simulink library "CommercialVehicleLibrary2G"  (R2021a)
settings: Solver=VariableStepAuto  StartTime=0.0  StopTime=10.0  RelTol=1e-3
values from neighbouring files (symbols this model uses):
  brake_input = [0   tmax ... (first row only)    [init_vehicle.m]    (also in run_Circle.m = [0  tmax; run_Coastdown.m = [0  2  tmax; run_DoubleLaneChangeDriver.m = [0   2  tmax; run_MaxAcc.m = [0  2  tmax)
  pose_t0 = [0 0 0 0]    [init_vehicle.m]    (also in run_Circle.m; run_Coastdown.m; run_DoubleLaneChangeDriver.m; run_MaxAcc.m)
  rdfname = 'TNO_FlatRoad.rdf'    [run_Circle.m]    (also in run_Coastdown.m; run_DoubleLaneChangeDriver.m; run_MaxAcc.m; run_Rollover.m)
  rdfname_inner = 'TNO_FlatRoad.rdf'    [run_Circle.m]    (also in run_Coastdown.m; run_DoubleLaneChangeDriver.m; run_MaxAcc.m; run_Rollover.m)
  steer_input = [0  tmax ... (first row only)    [init_vehicle.m]    (also in run_Circle.m = [0  2   10     13       tmax; run_Coastdown.m = [0 tmax; run_DoubleLaneChangeDriver.m = [0 tmax; run_MaxAcc.m = [0 tmax)
  throttle_input = [0         tmax ... (first row only)    [init_vehicle.m]    (also in run_Circle.m; run_Coastdown.m = [0        10         10.0001 tmax; run_DoubleLaneChangeDriver.m = [0        tmax; run_MaxAcc.m = [0        tmax)
  Vx = 0    [init_vehicle.m]    (also in run_Circle.m = Vx_kmh/3.6; run_Coastdown.m = Vx_kmh/3.6; run_DoubleLaneChangeDriver.m = Vx_kmh/3.6; run_MaxAcc.m)
  Vx_input = [0  tmax ... (first row only)    [init_vehicle.m]    (also in run_Circle.m; run_Coastdown.m = [0 tmax; run_DoubleLaneChangeDriver.m = [0 tmax; run_MaxAcc.m = [0 tmax)
undefined symbols (not defined in the file or in its folder): Drive, Floor, Fzstat, Fzstat1, Fzstat3, l, l_load1, l_load2, lbar, mass_load1, mass_load2, psi_semitrailer, rho, rim_Ixx, rim_Iyy, rim_mass, Steer, steer_path, tpfname, X, x_torsion, xcg, xcg1, xcg2, xcg_front, xcg_rear, xdrive1, xload1, xload2, xpos1, xref, xrev1, Xt0, Y, Yt0, Z
libraries: sm_lib x291, $bdroot x157, nesl_utility x143, vrlib x1
(part 1 of 12)
settings Model: Creator=ajayk  LastModifiedBy=ajayk
settings SolverCC: AlgebraicLoopSolver=TrustRegion
settings DebuggingCC: SFMachineParentedDataDiag=warning

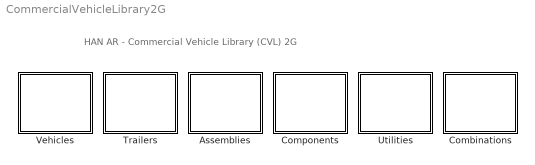
== system CommercialVehicleLibrary2G ==
  note: HAN AR - Commercial Vehicle Library (CVL) 2G
  Assemblies : Subsystem
      mask Display: disp('Assemblies')
  Combinations : Subsystem
      mask Display: disp('Combinations')
  Components : Subsystem
      mask Display: disp('Components')
  Trailers : Subsystem
      mask Display: disp('Trailers')
  Utilities : Subsystem
      mask Display: disp('Utilities')
  Vehicles : Subsystem
      mask Display: disp('Vehicles')

== system CommercialVehicleLibrary2G/Assemblies ==
  note: Axles
  note: Loads
  Cabin : Subsystem  mask(cabin with coil/air suspension){xref=xref+1.10, zref=1.20}
      mask prompts: xref "global X-coordinate cabin tip point [m]"; zref "global Z-coordinate cabin tip point [m]"
      mask Display: disp('Cabin')
  Dolly axle : Subsystem  mask(Axle with single tyres){xpos=0.7, tpfname='truck3.tpf', rdfname=rdfname, Vx=Vx, Fzstat=Fzstat}
      mask prompts: xpos "global X-coordinate wheelcentre [m]"; tpfname "tyre property file name [string]"; rdfname "road data file name  [string]"; Vx "initial velocity Vx [m/s]"; Fzstat "initial vertical axle load [N]"
      mask init:
      | Rtyre     = 0.546;
      | Cztyre    = 1.35e+006;
      | tyre_mass = 70;
      | 
      | zpos   =Rtyre - 0.5*Fzstat/Cztyre;
      | 
      | % dimensions
      | tw =2.0;  % [m], track_width
      | yd =1.0;  % [m], Y-distance bewteen dampers
      | ys =1.0;  % [m], Y-distance bewteen springs 
      | zrc=0.2;  % [m], height of roll centre wrt axle 
      |    
      | % damping/stiffness
      | Kspring = 394000;  % [N/m], spring stiffness (two per axle!)
      | Bdamper =  20000;  % [Ns/m] damper constant (two per axle!)
      | Kroll   =1516000;  % [Nm/rad] roll stiffness 
      |    
      | % mass/inertia
      | axle_mass = 400;  % [kg]
      | axle_Ixx  = 200; % [kgm2]
      | axle_Iyy  =  10;   % [kgm2]
      | axle_Izz  = 200; % [kgm2]
      |    
      | rim_mass= 55; % [kg]
      | rim_Ixx =  4; % [kgm2]
      | rim_Iyy =  6; % [kgm2] (including rotational inertia brake disk)
      | 
      | ld = 0.3;                     % loaded spring/damper length
      | ls = ld + 0.5*(Fzstat - 9.81*(axle_mass + 2*tyre_mass + 2*rim_mass))/Kspring;  % spring unloaded length
  Drive axle : Subsystem  mask(Driven axle with double tyres){xpos=xdrive1, tpfname='truck1.tpf', rdfname=rdfname, rdfname_inner=rdfname_inner, Vx=Vx, Fzstat=Fzstat3}
      mask prompts: xpos "global X-coordinate wheelcentre [m]"; tpfname "tyre property file name [string]"; rdfname "road data file name  [string]"; rdfname_inner "road data file name (inner)  [string]"; Vx "initial velocity Vx [m/s]"; Fzstat "initial vertical axle load [N]"
      mask init:
      | Rtyre     = 0.548;
      | Cztyre    = 1.13e+006;
      | tyre_mass = 62.7;
      | 
      | zpos = Rtyre - 0.25*Fzstat/Cztyre;
      | 
      | tw  =2.15;    % [m], track_width outer tyres
      | ywhl=0.35;   % [m], distance between double tyres
      | yd  =1.00;    % [m], Y-distance bewteen dampers
      | ys  =0.75;    % [m], Y-distance bewteen springs
      | zrc =0.30;   % [m], height of roll centre wrt axle centre 
      | 
      | % damping/stiffness
      | Kspring = 320000;    % [N/m], spring stiffness  (two per axle!)
      | Bdamper =  15000;    % [Ns/m], damper constant  (two per axle!)
      | Kroll   = 500000;    % [Nm/rad] roll stiffness 
      | 
      | % mass/inertia
      | axle_mass =1000;     % [kg] (excl. wheels/tyres!)
      | axle_Ixx  = 380;     % [kgm2]
      | axle_Iyy  =  10;     % [kgm2]
      | axle_Izz  = 380;     % [kgm2]
      |    
      | %rim
      | rim_mass= 50;        % [kg]
      | rim_Ixx =  3;        % [kgm2]
      | rim_Iyy =  5;        % [kgm2] (including rotational inertia brake disk)
      | 
      | ld = 0.3;            % loaded spring/damper length
      | ls = ld + 0.5*(Fzstat - 9.81*(axle_mass + 4*tyre_mass + 4*rim_mass))/Kspring;  % spring unloaded length
  Driveline : Subsystem  mask(Engine+gearbox){xref=xref-0.162, zref=0.58, param=DAF XEC + TC-Tronic (355 kW/2100 Nm)}
      mask prompts: xref "global X-coordinate engine ref. point [m]"; zref "global Z-coordinate engine ref. point [m]"; param "parameters"
      mask init:
      | % engine/gearbox: DAF XE355C / ZF 16S221
      | eng_power         = 355000;  % 355 kW
      | max_engine_torque = 2100;    % [Nm]
      | max_revs_rpm      = 1900;    % [rpm]
      | first_gear_ratio  = 16.41;   % [-]
      | final_drive_ratio =  3.07;   % [-]
      |  
      | % engine + gearbox mass (XEC +TC-tronic, DAF 51051/03-042 R. Liebrechts)
      | driveline_mass= 1800;       %[kg]
      | Ixx =  100;       %[kgm2]
      | Iyy =  900;       %[kgm2]
      | Izz =  900;       %[kgm2]
      | yrot=   0;        %[rad] rotation about Y-axis of inertial frame
      | xcg =  -0.25;     %[m], X-coordinate CG wrt rear engine mount ref. point
      | zcg =   0.30;     %[m], Z-coordinate CG wrt rear engine mount ref. point
      |  
      | omega_max=2*pi*max_revs_rpm/60;
      mask TypeOptions param: DAF XEC + TC-Tronic (355 kW/2100 Nm)
  Driver : Subsystem
  Steer axle : Subsystem  mask(Axle with single tyres and steering system){xpos=xref, tpfname='truck2b2.tpf', rdfname=rdfname, Vx=Vx, Fzstat=Fzstat1}
      mask prompts: xpos "global X-coordinate wheelcentre [m]"; tpfname "tyre property file name [string]"; rdfname "road data file name  [string]"; Vx "initial velocity Vx [m/s]"; Fzstat "initial vertical axle load [N]"
      mask init:
      | Rtyre    = 0.548;
      | Cztyre   = 1.19e+006;
      | tyre_mass= 62.7;
      | 
      | zpos=Rtyre - 0.5*Fzstat/Cztyre;
      | 
      | steerratio = 20; %[-], ratio steering wheel - front wheels
      |  
      | % dimensions
      | tw =2.0; 	% [m], track_width
      | zrc=0;    	% [m], height of roll centre wrt axle centerline   
      | yd =1.0; 	% [m], Y-distance bewteen dampers 
      | ys =0.85; 	% [m], Y-distance bewteen springs
      | 
      | % stiffness/damping
      | Kspring = 300000;  	% [N/m], spring stiffness (two per axle!)
      | Bdamper =  15000;  	% [Ns/m] damper constant  (two per axle!)
      | Kroll   = 200000;  	% [Nm/rad], roll stiffness 
      |    
      | % mass/inertia   
      | axle_mass = 475;    % [kg] (excl. wheels/tyres!)
      | axle_Ixx  = 200;	% [kgm2]
      | axle_Iyy  = 5;      % [kgm2]
      | axle_Izz  = 200;	% [kgm2]
      |    
      | %rim mass
      | rim_mass= 50; 	% [kg]
      | rim_Ixx =  3; 	% [kgm2]
      | rim_Iyy =  5; 	% [kgm2] (including rotational inertia brake disk)
      | 
      | ld = 0.3;       % loaded spring/damper length
      | ls = ld + 0.5*(Fzstat - 9.81*(axle_mass + 2*tyre_mass + 2*rim_mass))/Kspring;  % spring unloaded length
  Trailer axle : Subsystem  mask(Axle with single tyres){xpos=xpos1-xcg, tpfname='truck3.tpf', rdfname=rdfname, Vx=Vx, Fzstat=Fzstat}
      mask prompts: xpos "global X-coordinate wheelcentre [m]"; tpfname "tyre property file name [string]"; rdfname "road data file name  [string]"; Vx "initial velocity Vx [m/s]"; Fzstat "initial vertical axle load [N]"
      mask init: same as CommercialVehicleLibrary2G/Assemblies/Dolly axle
  Trailer load center : Subsystem  mask{xload=xload1, zload=1.3, mass_load=mass_load1, l_load=l_load1, w=2.5, rho=rho}
      mask prompts: xload "Global X-coordinate Center of Load [m]"; zload "Global Z-coordinate Application of Load [m]"; mass_load "mass [kg]"; l_load "length [m]"; w "width [m]"; rho "density [kg/m3]"
      mask init:
      | h=(mass_load)/(rho*w*(l_load));
      | zcg=0.5*h;
      | Ixx=(mass_load)*(w*w+h*h)/12;
      | Iyy=(mass_load)*((l_load)*(l_load)+h*h)/12;
      | Izz=(mass_load)*((l_load)*(l_load)+w*w)/12;
      mask Display: disp('Trailer center load ')
  Trailer load front : Subsystem  mask{xload=xload1, zload=1.3, mass_load=mass_load1, l_load=l_load1, w=2.5, rho=rho}
      mask prompts: xload "Global X-coordinate Center of Load [m]"; zload "Global Z-coordinate Application of Load [m]"; mass_load "mass [kg]"; l_load "length [m]"; w "width [m]"; rho "density [kg/m3]"
      mask init:
      | h=(mass_load)/(rho*w*(l_load));
      | zcg=0.5*h;
      | Ixx=(mass_load)*(w*w+h*h)/12;
      | Iyy=(mass_load)*((l_load)*(l_load)+h*h)/12;
      | Izz=(mass_load)*((l_load)*(l_load)+w*w)/12;
      mask Display: disp('Trailer front load ')
  Trailer load rear : Subsystem  mask{xload=xload2, zload=1.3, mass_load=mass_load2, l_load=l_load2, w=2.5, rho=rho}
      mask prompts: xload "Global X-coordinate Center of Load [m]"; zload "Global Z-coordinate Application of Load [m]"; mass_load "mass [kg]"; l_load "length [m]"; w "width [m]"; rho "density [kg/m3]"
      mask init:
      | h=(mass_load)/(rho*w*(l_load));
      | zcg=0.5*h;
      | Ixx=(mass_load)*(w*w+h*h)/12;
      | Iyy=(mass_load)*((l_load)*(l_load)+h*h)/12;
      | Izz=(mass_load)*((l_load)*(l_load)+w*w)/12;
      mask Display: disp('Trailer rear load ')
  Truck load : Subsystem  mask{xload=xload2, zload=1.3, mass_load=mass_load2, l_load=l_load2, w=2.5, rho=rho}
      mask prompts: xload "Global X-coordinate Center of Load [m]"; zload "Global Z-coordinate Application of Load [m]"; mass_load "mass [kg]"; l_load "length [m]"; w "width [m]"; rho "density [kg/m3]"
      mask init:
      | h=(mass_load)/(rho*w*(l_load));
      | zcg=0.5*h;
      | Ixx=(mass_load)*(w*w+h*h)/12;
      | Iyy=(mass_load)*((l_load)*(l_load)+h*h)/12;
      | Izz=(mass_load)*((l_load)*(l_load)+w*w)/12;
      mask Display: disp('Truck load ')

== system CommercialVehicleLibrary2G/Combinations ==
  note: Custom Combinations
  note: LZV Combinations
  LZV_A : Subsystem
      mask Display: disp('LZV - A')
  LZV_B : Subsystem
      mask Display: disp('LZV - B ')
  LZV_C : Subsystem
      mask Display: disp('LZV - C')
  LZV_D : Subsystem
      mask Display: disp('LZV - D')
  LZV_E : Subsystem
      mask Display: disp('LZV - E')
  LZV_F : Subsystem
      mask Display: disp('LZV - F')
  LZV_G : Subsystem
      mask Display: disp('LZV - G')
  "Tractor_semitrailer " : Subsystem
      mask Display: disp('Tractor + Semitrailer')
  Truck_dbtrailer : Subsystem
      mask Display: disp('Truck + DbTrailer')
  Truck_trailer : Subsystem
      mask Display: disp('Truck + Trailer')

== system CommercialVehicleLibrary2G/Components ==
  5th Wheel Joint : Subsystem
      mask Display: disp('5th Wheel Joint')
  Brake/Wheel_bearing : Subsystem  mask{Vx=Vx, radius=0.53}
      mask prompts: Vx "forward velocity (m/s)"; radius "tyre radius (m)"
  Braking system : Subsystem
  "Drawbar joint " : Subsystem
      mask Display: disp('Drawbar joint')
  MF Tyre L : Subsystem  Tag=SimMechanics Wheel + tyre  mask(SimMechanics_tyre){idtyre=1, inertia=[rim_mass rim_Ixx rim_Iyy], tpfname=tpfname, rdfname=rdfname, side_mode=(1xxx) left, cnt_mode=(x1xx) smooth road, dyn_mode=(xx1x) relaxation behaviour, mf_mode=(xxx4) combined, use_mode=1e8, disp_debug=off}
      mask prompts: idtyre "Tyre ID [integer]"; inertia "Rim inertia [3x real] mass (kg) Ixx Iyy (kgm2)"; tpfname "Tyre properties [string or struct]"; rdfname "Road data file [string]"; side_mode "Tyre side            :"; cnt_mode "Contact method :"; dyn_mode "Dynamics           :"; mf_mode "Slip forces          :"; use_mode "Optional: use mode (overrides pop-up) [current selection: 1114]"; disp_debug "Display debug messages"
      mask help:
      | Wheel + tyre model to be used in combination with the SimMechanics multibody toolbox.
      |
      | Tyre model version: MF-Tyre/MF-Swift 6.2
      | © 1996-2013 TNO, Helmond, The Netherlands
      |
      | MODIFIED VERSION by TU/e! (Igo Besselink)
      mask init:
      | % initialize parameters
      | % (required to overcome a bug in MATLAB 2006a: errors in a mask are not displayed,
      | %  and simulation is not ended. This check is carried out in s-function 
      | %  'chech_inertia_parameters' in the subsystem)
      | radius     = 1;
      | width      = 1;
      | belt_mass  = 1;
      | belt_Ixx   = 1;
      | belt_Iyy   = 1;
      | tyre_mass  = 1;
      | tyre_Ixx   = 1;
      | tyre_Iyy   = 1;
      | mass = 1;
      | Imat = [1 0 0; 0 1 0; 0 0 1];
      | 
      | % switch between tpf file or struct
      | if ischar(tpfname)
      |     typarr=zeros(300,1);
      |     tpfname_dummy=tpfname;
      |     if ~exist(tpfname_dummy)
      |         error('Tyre property file does not exist')
      |     end
      | elseif isstruct(tpfname)
      |     typarr=tno_tpf_struct2array(tpfname,idtyre);
      |     tpfname_dummy='';
      | else
      |     typarr=zeros(300,1);
      |     tpfname_dummy='';
      |     error(['Mask parameter ''Tyre property file'' should be supplied as string or structure for tyre ' num2str(idtyre)])
      | end
      | if ~exist(rdfname) && ~strcmp(rdfname,'')
      |     error('Road data file does not exist')
      | end
      | 
      | %initialisation script for SimMechanics
      | idroad=1;
      | 
      | %rim inertia as specified by the user in the GUI
      | rim_mass = inertia(1);
      | rim_Ixx  = inertia(2);
      | rim_Iyy  = inertia(3);
      | 
      | % check the use_mode of the model
      | if (abs(use_mode) > 4535 )
      |   iswtch=1000*side_mode+100*cnt_mode+10*(dyn_mode-1)+(mf_mode-1);
      | else
      |   iswtch=use_mode;
      | end
      | 
      | %get tyre inertia parameters from the tyre property file
      | if ischar(tpfname)
      |     [x,typarr]=dteval(tpfname_dummy,[1 2 3 4 5 6],1);
      | end
      | radius     = typarr(7);
      | width      = typarr(8);
      | belt_mass  = typarr(164);
      | belt_Ixx   = typarr(195);
      | belt_Iyy   = typarr(162);
      | tyre_mass  = typarr(190);
      | tyre_Ixx   = typarr(191);
      | tyre_Iyy   = typarr(192);
      | 
      | % display the use_mode of the model
      | if (disp_debug) disp(['Delft-Tyre ' num2str(idtyre) ' -> use_mode=' num2str(iswtch) ]); end
      | 
      | % check and calculate inertia of the rim_body
      | if  ( rim_mass <= 0 | rim_Ixx <= 0 | rim_Iyy <= 0 | tyre_mass <= 0 | tyre_Ixx <= 0 | tyre_Iyy <= 0 | belt_mass <= 0 | belt_Ixx <= 0 | belt_Iyy <= 0 )
      |   error('initialisation calculation results in a negative mass and/or inertia!') 
      |   disp_debug=1;
      | end
      | if  ( tyre_mass <= belt_mass | tyre_Ixx <= belt_Ixx | tyre_Iyy <= belt_Iyy  )
      |   error('initialisation calculation error: tyre belt mass/inertia > tyre mass/inertia!') 
      |   disp_debug=1;
      | end
      | 
      | if (disp_debug) 
      |   msg=[' wheel mass = ',num2str(rim_mass+tyre_mass),' kg'];
      |   disp(msg);
      |   msg=[' wheel Ixx  = ',num2str(rim_Ixx+tyre_Ixx),' kgm2'];
      |   disp(msg);
      |   msg=[' wheel Iyy  = ',num2str(rim_Iyy+tyre_Iyy),' kgm2'];
      |   disp(msg);
      |   msg=[' tyre mass  = ',num2str(tyre_mass),' kg (belt mass = ',num2str(belt_mass),' kg)' ];
      |   disp(msg);
      |   msg=[' tyre Ixx   = ',num2str(tyre_Ixx) ,' kgm2 (belt Ixx  = ',num2str(belt_Ixx) ,' kgm2)'];
      |   disp(msg);
      |   msg=[' tyre Iyy   = ',num2str(tyre_Iyy) ,' kgm2 (belt Iyy  = ',num2str(belt_Iyy) ,' kgm2)'];
      |   disp(msg);
      | end
      | 
      | % calculate the mass of the wheelbody in the MBS environment 
      | %   normally           : rim + tyre
      | %   rigid ring dynamics: rim + part of tyre (and separate rigid body inside tyre model)
      | dynmod=iswtch-100*floor(iswtch/100);
      | if (dynmod/10 >= 3) 
      |   %rigid ring dynamics switched on
      |   wheelbody_mass = rim_mass + tyre_mass - belt_mass;
      |   wheelbody_Ixx  = rim_Ixx  + tyre_Ixx  - belt_Ixx;
      |   wheelbody_Iyy  = rim_Iyy  + tyre_Iyy  - belt_Iyy;
      | else
      |   %rigid ring dynamics switched off
      |   wheelbody_mass = rim_mass + tyre_mass;
      |   wheelbody_Ixx  = rim_Ixx  + tyre_Ixx;
      |   wheelbody_Iyy  = rim_Iyy  + tyre_Iyy;
      | end
      | 
      | mass = wheelbody_mass;
      | Imat = [wheelbody_Ixx 0 0; 0 wheelbody_Iyy 0; 0 0 wheelbody_Ixx];
      | 
      | fliplr = 0;
      | % CHANGE GEOMETRY ORIENTATION IF WHEEL IS ON RIGHT SIDE
      | if (side_mode == 2)
      |     fliplr=1;
      |     %disp(['Tyre ID = ' num2str(idtyre) ', fliplr = ' num2str(fliplr)]);
      | end
      mask Help: eval('DTOpenHelp(506)')
      mask TypeOptions side_mode: (1xxx) left | (2xxx) right | (3xxx) symmetric
      mask Callback side_mode:
      | promtstr = get_param(gcb,'MaskPromptString');
      | index = find(double(promtstr)==124);
      | maskval = get_param(gcb,'MaskValues');
      | new_mode = [maskval{5}(2) maskval{6}(3) maskval{7}(4) maskval{8}(5)];
      | newpromtstr = [promtstr(1:index(8)) ['Optional: use mode (overrides pop-up) [current selection: ' new_mode ']'] promtstr(index(9):end)];
      | set_param(gcb,'MaskPromptString',newpromtstr);
      mask TypeOptions cnt_mode: (x1xx) smooth road | (x2xx) smooth road (motorcycle: circular cross section) | (x3xx) moving road | (x4xx) 2D short wavelength road contact | (x5xx) 3D short wavelength road contact
      mask Callback cnt_mode:
      | promtstr = get_param(gcb,'MaskPromptString');
      | index = find(double(promtstr)==124);
      | maskval = get_param(gcb,'MaskValues');
      | new_mode = [maskval{5}(2) maskval{6}(3) maskval{7}(4) maskval{8}(5)];
      | newpromtstr = [promtstr(1:index(8)) ['Optional: use mode (overrides pop-up) [current selection: ' new_mode ']'] promtstr(index(9):end)];
      | set_param(gcb,'MaskPromptString',newpromtstr);
      mask TypeOptions dyn_mode: (xx0x) steady-state | (xx1x) relaxation behaviour | (xx2x) relaxation behaviour - non-linear | (xx3x) rigid ring | (xx4x) rigid ring + initial statics
      mask Callback dyn_mode:
      | promtstr = get_param(gcb,'MaskPromptString');
      | index = find(double(promtstr)==124);
      | maskval = get_param(gcb,'MaskValues');
      | new_mode = [maskval{5}(2) maskval{6}(3) maskval{7}(4) maskval{8}(5)];
      | newpromtstr = [promtstr(1:index(8)) ['Optional: use mode (overrides pop-up) [current selection: ' new_mode ']'] promtstr(index(9):end)];
      | set_param(gcb,'MaskPromptString',newpromtstr);
      mask TypeOptions mf_mode: (xxx0) none | (xxx1) longitudinal | (xxx2) lateral | (xxx3) uncombined | (xxx4) combined | (xxx5) combined+turnslip
      mask Callback mf_mode:
      | promtstr = get_param(gcb,'MaskPromptString');
      | index = find(double(promtstr)==124);
      | maskval = get_param(gcb,'MaskValues');
      | new_mode = [maskval{5}(2) maskval{6}(3) maskval{7}(4) maskval{8}(5)];
      | newpromtstr = [promtstr(1:index(8)) ['Optional: use mode (overrides pop-up) [current selection: ' new_mode ']'] promtstr(index(9):end)];
      | set_param(gcb,'MaskPromptString',newpromtstr);
  MF Tyre R : Subsystem  Tag=SimMechanics Wheel + tyre  mask(SimMechanics_tyre){idtyre=2, inertia=[rim_mass rim_Ixx rim_Iyy], tpfname=tpfname, rdfname=rdfname, side_mode=(2xxx) right, cnt_mode=(x1xx) smooth road, dyn_mode=(xx1x) relaxation behaviour, mf_mode=(xxx4) combined, use_mode=1e8, disp_debug=off}
      mask prompts: idtyre "Tyre ID [integer]"; inertia "Rim inertia [3x real] mass (kg) Ixx Iyy (kgm2)"; tpfname "Tyre properties [string or struct]"; rdfname "Road data file [string]"; side_mode "Tyre side            :"; cnt_mode "Contact method :"; dyn_mode "Dynamics           :"; mf_mode "Slip forces          :"; use_mode "Optional: use mode (overrides pop-up) [current selection: 2114]"; disp_debug "Display debug messages"
      mask help:
      | Wheel + tyre model to be used in combination with the SimMechanics multibody toolbox.
      |
      | Tyre model version: MF-Tyre/MF-Swift 6.2
      | © 1996-2013 TNO, Helmond, The Netherlands
      |
      | MODIFIED VERSION by TU/e! (Igo Besselink)
      mask init: same as CommercialVehicleLibrary2G/Components/MF Tyre L
      mask Help: eval('DTOpenHelp(506)')
      mask TypeOptions side_mode: (1xxx) left | (2xxx) right | (3xxx) symmetric
      mask Callback side_mode:
      | promtstr = get_param(gcb,'MaskPromptString');
      | index = find(double(promtstr)==124);
      | maskval = get_param(gcb,'MaskValues');
      | new_mode = [maskval{5}(2) maskval{6}(3) maskval{7}(4) maskval{8}(5)];
      | newpromtstr = [promtstr(1:index(8)) ['Optional: use mode (overrides pop-up) [current selection: ' new_mode ']'] promtstr(index(9):end)];
      | set_param(gcb,'MaskPromptString',newpromtstr);
      mask TypeOptions cnt_mode: (x1xx) smooth road | (x2xx) smooth road (motorcycle: circular cross section) | (x3xx) moving road | (x4xx) 2D short wavelength road contact | (x5xx) 3D short wavelength road contact
      mask Callback cnt_mode:
      | promtstr = get_param(gcb,'MaskPromptString');
      | index = find(double(promtstr)==124);
      | maskval = get_param(gcb,'MaskValues');
      | new_mode = [maskval{5}(2) maskval{6}(3) maskval{7}(4) maskval{8}(5)];
      | newpromtstr = [promtstr(1:index(8)) ['Optional: use mode (overrides pop-up) [current selection: ' new_mode ']'] promtstr(index(9):end)];
      | set_param(gcb,'MaskPromptString',newpromtstr);
      mask TypeOptions dyn_mode: (xx0x) steady-state | (xx1x) relaxation behaviour | (xx2x) relaxation behaviour - non-linear | (xx3x) rigid ring | (xx4x) rigid ring + initial statics
      mask Callback dyn_mode:
      | promtstr = get_param(gcb,'MaskPromptString');
      | index = find(double(promtstr)==124);
      | maskval = get_param(gcb,'MaskValues');
      | new_mode = [maskval{5}(2) maskval{6}(3) maskval{7}(4) maskval{8}(5)];
      | newpromtstr = [promtstr(1:index(8)) ['Optional: use mode (overrides pop-up) [current selection: ' new_mode ']'] promtstr(index(9):end)];
      | set_param(gcb,'MaskPromptString',newpromtstr);
      mask TypeOptions mf_mode: (xxx0) none | (xxx1) longitudinal | (xxx2) lateral | (xxx3) uncombined | (xxx4) combined | (xxx5) combined+turnslip
      mask Callback mf_mode:
      | promtstr = get_param(gcb,'MaskPromptString');
      | index = find(double(promtstr)==124);
      | maskval = get_param(gcb,'MaskValues');
      | new_mode = [maskval{5}(2) maskval{6}(3) maskval{7}(4) maskval{8}(5)];
      | newpromtstr = [promtstr(1:index(8)) ['Optional: use mode (overrides pop-up) [current selection: ' new_mode ']'] promtstr(index(9):end)];
      | set_param(gcb,'MaskPromptString',newpromtstr);
  Tractor_torsion : Subsystem
      settings: PortSchema="{\"entries\":[{\"content\":{\"sides\":[{\"content\":{\"connectorIds\":[\"LConn1\"]},\"type\":\"ConnectorPlacement.EquallySpacedRectSide\",\"uuid\":\"b43c74bd-af15-4ffb-863b-6a132848d787\"},{\"content\":{\"connectorIds\":[\"RConn1\"],\"side\":\"RIGHT\"},\"type\":\"ConnectorPlacement.EquallySpacedRectSide\",\"uuid\":\"8ef5ae9f-2f99-4b38-816f-c2fb0756fe1b\"},{\"content\":{\"connectorIds\":[\"Out1\"],\"side\":\"TOP\"},\"type\":\"ConnectorPlacement.EquallySpacedRectSide\",\"uuid\":\"649c363b-e78d-45fa-ac8c-bda3eda724e3\"}]},\"type\":\"ConnectorPlacement.EquallySpacedConnector\",\"uuid\":\"06fb9ebd-5177-4420-93bb-82569f181fb4\"}],\"packageUris\":[\"http://schema.mathworks.com/mf0/Connector/R2020b\"],\"version\":\"1.0\"}"
  Trailer_torsion : Subsystem
      settings: PortSchema="{\"entries\":[{\"content\":{\"sides\":[{\"content\":{\"connectorIds\":[\"LConn1\"]},\"type\":\"ConnectorPlacement.EquallySpacedRectSide\",\"uuid\":\"b43c74bd-af15-4ffb-863b-6a132848d787\"},{\"content\":{\"connectorIds\":[\"RConn1\"],\"side\":\"RIGHT\"},\"type\":\"ConnectorPlacement.EquallySpacedRectSide\",\"uuid\":\"8ef5ae9f-2f99-4b38-816f-c2fb0756fe1b\"},{\"content\":{\"connectorIds\":[\"Out1\"],\"side\":\"TOP\"},\"type\":\"ConnectorPlacement.EquallySpacedRectSide\",\"uuid\":\"649c363b-e78d-45fa-ac8c-bda3eda724e3\"}]},\"type\":\"ConnectorPlacement.EquallySpacedConnector\",\"uuid\":\"06fb9ebd-5177-4420-93bb-82569f181fb4\"}],\"packageUris\":[\"http://schema.mathworks.com/mf0/Connector/R2020b\"],\"version\":\"1.0\"}"
  Truck_torsion : Subsystem
      settings: PortSchema="{\"entries\":[{\"content\":{\"sides\":[{\"content\":{\"connectorIds\":[\"LConn1\"]},\"type\":\"ConnectorPlacement.EquallySpacedRectSide\",\"uuid\":\"b43c74bd-af15-4ffb-863b-6a132848d787\"},{\"content\":{\"connectorIds\":[\"RConn1\"],\"side\":\"RIGHT\"},\"type\":\"ConnectorPlacement.EquallySpacedRectSide\",\"uuid\":\"8ef5ae9f-2f99-4b38-816f-c2fb0756fe1b\"},{\"content\":{\"connectorIds\":[\"Out1\"],\"side\":\"TOP\"},\"type\":\"ConnectorPlacement.EquallySpacedRectSide\",\"uuid\":\"649c363b-e78d-45fa-ac8c-bda3eda724e3\"}]},\"type\":\"ConnectorPlacement.EquallySpacedConnector\",\"uuid\":\"06fb9ebd-5177-4420-93bb-82569f181fb4\"}],\"packageUris\":[\"http://schema.mathworks.com/mf0/Connector/R2020b\"],\"version\":\"1.0\"}"

== system CommercialVehicleLibrary2G/Trailers ==
  Dolly : Subsystem  mask(semitrailer (3 non-steered axles)){xref=-8.35, lbar=3.50, Fzstat=6700*9.81}
      mask prompts: xref "Global X-coordinate pin coupling [m]"; lbar "Distance pin coupling to dolly centre [m]"; Fzstat "Initial vertical axle load [N]"
      mask init:
      | %Connection Body Properties
      | xcg = xref-lbar;             % [m],C.G. of connection body wrt global-X coordinate
      | 
      | l=1.6;
      | w=0.8;
      | h=0.2;
      | chassis_mass= 500;                           % [kg] 
      | chassis_Ixx = chassis_mass*(w*w+h*h)/12;     % [kgm2]
      | chassis_Iyy = chassis_mass*(l*l+h*h)/12;     % [kgm2]
      | chassis_Izz = chassis_mass*(l*l+w*w)/12;     % [kgm2]
  "Drawbar Trailer - 2 axle " : Subsystem  mask(semitrailer (3 non-steered axles)){xref=-15.06+1, l_chassis=7.82, lbar=2.0, mass_empty=3900, mass_load=13600, rho=350, Fzstat=8500*9.81}
      mask prompts: xref "Global X-coordinate pin coupling [m]"; l_chassis "Trailer chassis length [m]"; lbar "Distance front trailer to pin coupler [m]"; mass_empty "Mass of empty trailer [kg]"; mass_load "Mass of load [kg]"; rho "Density of load [kg/m3]"; Fzstat "Initial vertical axle load [N]"
      mask init:
      | %Drawbar Properties
      | zbar=0.6;
      | drawbar_mass=400;                 % [kg]
      | 
      | %Trailer Properties
      | xcg2=-0.5*lbar-0.5*l_chassis;        % [m]
      | 
      | l=l_chassis;
      | w=1.5;
      | h=0.3;
      | chassis_mass= (mass_empty - 2*650 - drawbar_mass);  % [kg] 
      | chassis_Ixx = chassis_mass*(w*w+h*h)/12;            % [kgm2]
      | chassis_Iyy = chassis_mass*(l*l+h*h)/12;            % [kgm2]
      | chassis_Izz = chassis_mass*(l*l+w*w)/12;            % [kgm2]
      | 
      | %Position of the first and second trailer axle from the chassis CG
      | xpos1= xcg2 -0.06 +0.9;
      | xpos2= xcg2 -0.06 -0.9;
  "Drawbar Trailer - 3 axle " : Subsystem  mask(semitrailer (3 non-steered axles)){xref=-9.6, l_chassis=10.0, lbar=2.0, mass_empty=6000, mass_load=22000, rho=350, Fzstat=9100*9.81}
      mask prompts: xref "Global X-coordinate pin coupling [m]"; l_chassis "Trailer chassis length [m]"; lbar "Distance front trailer to pin coupler [m]"; mass_empty "Mass of empty trailer [kg]"; mass_load "Mass of load [kg]"; rho "Density of load [kg/m3]"; Fzstat "Initial vertical axle load [N]"
      mask init:
      | %Drawbar Properties
      | zbar=0.6;
      | drawbar_mass=500;                 % [kg]
      | 
      | %Trailer Properties
      | xcg2=xref-lbar-l_chassis/2;        % [m]
      | 
      | l=l_chassis;
      | w=1.5;
      | h=0.3;
      | chassis_mass= (mass_empty - 3*650 - drawbar_mass);  % [kg] 
      | chassis_Ixx = chassis_mass*(w*w+h*h)/12;            % [kgm2]
      | chassis_Iyy = chassis_mass*(l*l+h*h)/12;            % [kgm2]
      | chassis_Izz = chassis_mass*(l*l+w*w)/12;            % [kgm2]
      | 
      | %Position of the first and second trailer axle
      | xpos1= xcg2 -0.05 +1.8;
      | xpos2= xcg2 -0.05;
      | xpos3= xcg2 -0.05 -1.8;
  Semitrailer : Subsystem  mask(semitrailer (3 non-steered axles)){xref=-3.06, xaxle2=8.475, lchassis=12.0, x5th=1.6, mass_empty=5000, mass_load=14500, rho=350, Fzstat=6400*9.81, lbdouble=0, psi_semitrailer=pose_t0(4)}
      mask prompts: xref "Global X-coordinate 5th wheel [m]"; xaxle2 "Distance 5th wheel to second semitrailer axle [m]"; lchassis "Semitrailer chassis length [m]"; x5th "Distance front trailer to 5th wheel [m]"; mass_empty "Mass of empty semitrailer [kg]"; mass_load "Mass of load [kg]"; rho "Density of load [kg/m3]"; Fzstat "Initial vertical axle load [N]"; lbdouble "B-double load length reduction (rear side) [m]"; psi_semitrailer "Articulation angle (t=0) [rad]"
      mask init:
      | %Semitrailer chassis
      | xcg1  = xref+x5th-0.25*lchassis;            % [m], Center of the first semitrailer chassis wrt global axis system
      | xcg2  = xref+x5th-0.75*lchassis;            % [m], Center of the second semitrailer chassis wrt global axis system
      | xrev1 = xref+x5th-0.5*lchassis;             % [m], Position of torsional spring wrt global axis system
      | 
      | l=0.5*lchassis;
      | w=1.5;
      | h=0.3;
      | chassis_mass= (mass_empty-3*650)/2;         % [kg] 
      | chassis_Ixx = chassis_mass*(w*w+h*h)/12;    % [kgm2]
      | chassis_Iyy = chassis_mass*(l*l+h*h)/12;    % [kgm2]
      | chassis_Izz = chassis_mass*(l*l+w*w)/12;    % [kgm2]
      | 
      | %Loading
      | l_load1 = 0.5*lchassis;
      | l_load2 = 0.5*lchassis-lbdouble;
      | xload1  = xref+x5th-0.5*l_load1;             % [m], Global X-coordinate center of load1
      | xload2  = xref+x5th-0.5*l_load2-l_load1;     % [m], Global X-coordinate center of load2
      | 
      | mass_load1 = l_load1/(l_load1+l_load2)*mass_load;
      | mass_load2 = l_load2/(l_load1+l_load2)*mass_load;
  "Trailer - 2 axle " : Subsystem  mask(semitrailer (3 non-steered axles)){xref=-8.03, xtrailer=5.42, l_chassis=7.82, lturn=1.2, lbar=2.7, mass_empty=5000, mass_load=10000, rho=250, Fzstat=7500*9.81}
      mask prompts: xref "Global X-coordinate pin coupling [m]"; xtrailer "Distance between the first and second trailer axle [m]"; l_chassis "Trailer chassis length [m]"; lturn "Distance front trailer to front axle rotation point [m]"; lbar "Draw bar length [m]"; mass_empty "Mass of empty trailer [kg]"; mass_load "Mass of load [kg]"; rho "Density of load [kg/m3]"; Fzstat "Initial vertical axle load [N]"
      mask init:
      | %Drawbar Properties
      | %Trailer chassis
      | xcg1  = xref -lbar +lturn - 0.25*l_chassis;    % [m]
      | xcg2  = xref -lbar +lturn - 0.75*l_chassis;    % [m]
      | xrev1 = xref -lbar +lturn - 0.50*l_chassis;    % [m]% [m], Position of torsional spring wrt global axis system
      | 
      | l=0.5*l_chassis;
      | w=1.5;
      | h=0.3;
      | chassis_mass= (mass_empty-2*650)/2;         % [kg] 
      | chassis_Ixx = chassis_mass*(w*w+h*h)/12;    % [kgm2]
      | chassis_Iyy = chassis_mass*(l*l+h*h)/12;    % [kgm2]
      | chassis_Izz = chassis_mass*(l*l+w*w)/12;    % [kgm2]
      | 
      | %Position of the 1st,2nd and 3rd trailer axle
      | xpos1 = xref -lbar;                         % [m], Global X-coordinate wheelcentre1
      | xpos2 = xpos1-xtrailer;                     % [m], Global X-coordinate wheelcentre2
      | xpos3 = xpos2-1.4;                          % [m], Global X-coordinate wheelcentre3
  "Trailer - 3 axle " : Subsystem  mask(semitrailer (3 non-steered axles)){xref=-10.0, xtrailer=5, l_chassis=10, lturn=1.2, lbar=2.7, mass_empty=6000, mass_load=22000, rho=350, Fzstat=9333*9.81}
      mask prompts: xref "Global X-coordinate pin coupling [m]"; xtrailer "Distance between the first and second trailer axle [m]"; l_chassis "Trailer chassis length [m]"; lturn "Distance front trailer to front axle rotation point [m]"; lbar "Draw bar length [m]"; mass_empty "Mass of empty trailer [kg]"; mass_load "Mass of load [kg]"; rho "Density of load [kg/m3]"; Fzstat "Initial vertical axle load [N]"
      mask init: same as CommercialVehicleLibrary2G/Trailers/Trailer - 2 axle 

== system CommercialVehicleLibrary2G/Utilities ==
  note: MF Tyre Inputs
  note: Truck Workspaces
  note: Trailer Workspaces
  Differentiator/filter : Subsystem  mask{ts=0.05}
      mask prompts: ts "response_time"
      mask init:
      | c=(3*pi/ts)^2;
  Non-moving road : Subsystem  Tag=Non-moving road  mask{dummy=off}
  Scaling factors : Subsystem  Tag=Scaling factors  mask{LMUX=1, LKX=1, LMUY=1, LKY=1, LKYC=1, LTR=1, LKZC=1}
      mask prompts: LMUX "longitudinal friction"; LKX "longitudinal slip stiffness"; LMUY "lateral fiction"; LKY "cornering stiffness"; LKYC "camber stiffness"; LTR "pneumatic trail"; LKZC "camber torque stiffness"
  To_workspace_dolly : Subsystem
      mask Display: disp('Workspace - Dolly')
  To_workspace_drawbar_trailer_2axle : Subsystem
      mask Display: disp('Workspace - Drawbar Trailer 2axle')
  To_workspace_drawbar_trailer_3axle : Subsystem
      mask Display: disp('Workspace - Drawbar Trailer 3axle')
  To_workspace_semitrailer : Subsystem
      mask Display: disp('Workspace - Semitrailer')
  To_workspace_tractor : Subsystem
      mask Display: disp('Workspace - Tractor')
  To_workspace_trailer_2axle : Subsystem
      mask Display: disp('Workspace - Trailer 2axle')
  To_workspace_trailer_3axle : Subsystem
      mask Display: disp('Workspace - Trailer 3axle')
  To_workspace_truck_2axle : Subsystem
      mask Display: disp('Workspace - Truck 2axle')
  To_workspace_truck_3axle : Subsystem
      mask Display: disp('Workspace - Truck 3axle')
  To_workspace_truck_4axle : Subsystem
      mask Display: disp('Workspace - Truck 4 axle')
  World : Subsystem

== system CommercialVehicleLibrary2G/Vehicles ==
  Rigid Truck - 2 axles : Subsystem  mask{xref=0, xaxle=5.9, l_load=7.5, mass_load=10000, rho=250, Fzstat1=7500*9.81, Fzstat2=11500*9.81, Xt0=pose_t0(1), Yt0=pose_t0(2), Psit0=pose_t0(3)}
      mask prompts: xref "Global X-coordinate front axle [m]"; xaxle "Distance front axle to rear axle [m]"; l_load "Length of load [m]"; mass_load "Mass of Load [kg]"; rho "Density of load [kg/m3]"; Fzstat1 "Steer Axle Initial Vertical Axle Load [N]"; Fzstat2 "Drive Axle Initial Vertical Axle Load [N]"; Xt0 "Global X-position front axle tractor [m]"; Yt0 "Global Y-position front axle tractor [m]"; Psit0 "Heading angle tractor [rad]"
      mask init:
      | % Torsional joint 
      | x_torsion = xref-1.3;   % [m],X-coordinate torsional joint wrt reference point
      | 
      | % Front part of vehicle chassis
      | l1=2.6;
      | w1=1.5;
      | h1=0.3;
      | xcg_front  = xref;   % [m],X-coordinate C.G. wrt reference point
      | front_mass = 1349;   % [kg]
      | front_Ixx  = front_mass*(w1*w1+h1*h1)/12;    % [kgm2]
      | front_Iyy  = front_mass*(l1*l1+h1*h1)/12;    % [kgm2]
      | front_Izz  = front_mass*(l1*l1+w1*w1)/12;    % [kgm2]
      | 
      | % Rear part of vehicle chassis
      | l2=l_load-0.3;   % load starts 1 m after front axle, torsional joint 1.3 m behind front axle
      | w2=1.5;
      | h2=0.3;
      | xcg_rear  = xref-1.3 - 0.5*l2;          % [m], global X-coordinate CG 
      | rear_mass = 2400;                       % [kg] 
      | rear_Ixx  = rear_mass*(w2*w2+h2*h2)/12;    % [kgm2]
      | rear_Iyy  = rear_mass*(l2*l2+h2*h2)/12;    % [kgm2]
      | rear_Izz  = rear_mass*(l2*l2+w2*w2)/12;    % [kgm2]
      | 
      | % Load Location
      | xload = xref -1 - 0.5*l_load;          % [m] global X-coordinate center of load
      mask DialogControl IniPos Prompt: Initial vehicle position (At t=0 sec.)
  Rigid Truck - 3 axles : Subsystem  mask{xref=0, xaxle=5.0, l_load=7.82, mass_load=15000, rho=350, Fzstat1=7500*9.81, Fzstat2=9250*9.81, Fzstat3=9250*9.81, Xt0=pose_t0(1), Yt0=pose_t0(2), Psit0=pose_t0(3)}
      mask prompts: xref "Global X-coordinate front axle [m]"; xaxle "Distance front axle to rear axle [m]"; l_load "Length of load [m]"; mass_load "Mass of Load [kg]"; rho "Density of load [kg/m3]"; Fzstat1 "Steer Axle Initial Vertical Axle Load [N]"; Fzstat2 "Drive Axle1 Initial Vertical Axle Load [N]"; Fzstat3 "Drive Axle2 Initial Vertical Axle Load [N]"; Xt0 "Global X-position front axle tractor [m]"; Yt0 "Global Y-position front axle tractor [m]"; Psit0 "Heading angle tractor [rad]"
      mask init:
      | % Torsional joint 
      | x_torsion = xref-1.3;   % [m],X-coordinate torsional joint wrt reference point
      | 
      | % Front part of vehicle chassis
      | l1=2.6;
      | w1=1.5;
      | h1=0.3;
      | xcg_front  = xref;   % [m],X-coordinate C.G. wrt reference point
      | front_mass = 1349-10;   % [kg]
      | front_Ixx  = front_mass*(w1*w1+h1*h1)/12;    % [kgm2]
      | front_Iyy  = front_mass*(l1*l1+h1*h1)/12;    % [kgm2]
      | front_Izz  = front_mass*(l1*l1+w1*w1)/12;    % [kgm2]
      | 
      | % Rear part of vehicle chassis
      | l2=l_load-0.3;   % load starts 1 m after front axle, torsional joint 1.3 m behind front axle
      | w2=1.5;
      | h2=0.3;
      | xcg_rear  = xref-1.3 - 0.5*l2;          % [m], global X-coordinate CG 
      | rear_mass = 2950+10;                       % [kg] 
      | rear_Ixx  = rear_mass*(w2*w2+h2*h2)/12;    % [kgm2]
      | rear_Iyy  = rear_mass*(l2*l2+h2*h2)/12;    % [kgm2]
      | rear_Izz  = rear_mass*(l2*l2+w2*w2)/12;    % [kgm2]
      | 
      | % Load Location
      | xload = xref -1 - 0.5*l_load;          % [m] global X-coordinate center of load
      mask DialogControl IniPos Prompt: Initial vehicle position (At t=0 sec.)
  Rigid Truck - 4 axles : Subsystem  mask{xref=0, xaxle=5.1, l_chassis=12, l_load=9.6, mass_load=19000, rho=350, Fzstat1=7500*9.81, Fzstat2=7500*9.81, Fzstat3=8500*9.81, Fzstat4=8500*9.81, conf=Steer-Steer-Drive-Drive, Xt0=pose_t0(1), Yt0=pose_t0(2), Psit0=pose_t0(3)}
      mask prompts: xref "Global X-coordinate front axle [m]"; xaxle "Distance front axle to rear axle [m]"; l_chassis "Total truck length [m]"; l_load "Length of load [m]"; mass_load "Mass of Load [kg]"; rho "Density of load [kg/m3]"; Fzstat1 "Steer Axle 1 Initial Vertical Axle Load [N]"; Fzstat2 "Steer Axle 2 Initial Vertical Axle Load [N]"; Fzstat3 "Drive Axle 1 Initial Vertical Axle Load [N]"; Fzstat4 "Drive Axle 2 Initial Vertical Axle Load [N]"; conf "Configuration"; Xt0 "Global X-position front axle tractor [m]"; Yt0 "Global Y-position front axle tractor [m]"; Psit0 "Heading angle tractor [rad]"
      mask init:
      | % Torsional joint 
      | x_torsion = xref-1.3;   % [m],X-coordinate torsional joint wrt reference point
      | 
      | % Front part of vehicle chassis
      | l1=2.6;
      | w1=1.5;
      | h1=0.3;
      | xcg_front  = xref;   % [m],X-coordinate C.G. wrt reference point
      | front_mass = 1349-30;   % [kg]
      | front_Ixx  = front_mass*(w1*w1+h1*h1)/12;    % [kgm2]
      | front_Iyy  = front_mass*(l1*l1+h1*h1)/12;    % [kgm2]
      | front_Izz  = front_mass*(l1*l1+w1*w1)/12;    % [kgm2]
      | 
      | % Rear part of vehicle chassis
      | l2=l_chassis-2.6;   %  torsional joint 1.3 m behind front axle + 1.4 m vehicle ahead of front axle
      | w2=1.5;
      | h2=0.3;
      | xcg_rear  = xref-1.3 - 0.5*l2;          % [m], global X-coordinate CG 
      | rear_mass = 4250+30;                       % [kg] 
      | rear_Ixx  = rear_mass*(w2*w2+h2*h2)/12;    % [kgm2]
      | rear_Iyy  = rear_mass*(l2*l2+h2*h2)/12;    % [kgm2]
      | rear_Izz  = rear_mass*(l2*l2+w2*w2)/12;    % [kgm2]
      | 
      | if (conf==1)
      |   %2nd steer axle is 2nd axle
      |   xsteer2=xref-xaxle;
      |   xdrive1=xref-xaxle-1.40;
      |   xdrive2=xref-xaxle-2.80;
      |   steer_ratio = 2.1/(xaxle+2.1);
      | end
      | 
      | if (conf==2)
      |   %2nd steer axle is 4th axle
      |   xsteer2=xref-xaxle-2.80;
      |   xdrive1=xref-xaxle;
      |   xdrive2=xref-xaxle-1.40;
      |   steer_ratio = -2.1/(xaxle+0.7);
      | end
      | 
      | % Load Location
      | xload = xref - 1 - 0.5*l_load;         % [m] global X-coordinate center of load
      mask TypeOptions conf: Steer-Steer-Drive-Drive | Steer-Drive-Drive-Steer
      mask DialogControl IniPos Prompt: Initial vehicle position (At t=0 sec.)
  Tractor : Subsystem  mask{xref=0, xrear=-3.80, Fzstat1=7500*9.81, Fzstat2=11500*9.81, Xt0=pose_t0(1), Yt0=pose_t0(2), Psit0=pose_t0(3)}
      mask prompts: xref "Global X-coordinate front axle [m]"; xrear "X-coordinate rear axle (relative to front) [m]"; Fzstat1 "Steer Axle Initial Vertical Axle Load [N]"; Fzstat2 "Drive Axle Initial Vertical Axle Load [N]"; Xt0 "Global X-position front axle tractor [m]"; Yt0 "Global Y-position front axle tractor [m]"; Psit0 "Heading angle tractor [rad]"
      mask init:
      | % Torsional joint 
      | x_torsion = xref-1.3;   % [m],X-coordinate torsional joint wrt reference point
      | 
      | % Front part of vehicle chassis
      | l1=2.6;
      | w1=1.0;
      | h1=0.3;
      | xcg_front  = xref;   % [m],X-coordinate C.G. wrt reference point
      | front_mass = 1349;   % [kg]
      | front_Ixx  = front_mass*(w1*w1+h1*h1)/12;    % [kgm2]
      | front_Iyy  = front_mass*(l1*l1+h1*h1)/12;    % [kgm2]
      | front_Izz  = front_mass*(l1*l1+w1*w1)/12;    % [kgm2]
      | 
      | % Rear part of vehicle chassis
      | l2=3.3;
      | w2=1.0;
      | h2=0.3;
      | xcg_rear  = xref-1.3 - 0.5*l2;          % [m], global X-coordinate CG 
      | rear_mass = 400;                       % [kg] 
      | rear_Ixx  = rear_mass*(w2*w2+h2*h2)/12;    % [kgm2]
      | rear_Iyy  = rear_mass*(l2*l2+h2*h2)/12;    % [kgm2]
      | rear_Izz  = rear_mass*(l2*l2+w2*w2)/12;    % [kgm2]
      mask DialogControl IniPos Prompt: Initial vehicle position (At t=0 sec.)

== system CommercialVehicleLibrary2G/Assemblies/Cabin ==
  Brick Solid : sm_lib/Body Elements/Brick Solid  GraphicAmbientColor=[0.15 0.15 0.15 1.0]  BasedOnType=Density  BrickDimensions=[1 1 1]  BrickDimensionUnits=m  CenterOfMass=[0 0 0]  CenterOfMassUnits=m  GraphicDiffuseColor=[1 1 1]  Density=1000  DensityUnits=kg/m^3  DoExposeReferenceFrame=on  GraphicEmissiveColor=[0.0 0.0 0.0 1.0]  ExportEntireGeometry=off  SerializedFrames=<Frames><Frame><Id>Frame1</Id><Value><Name>F1</Name><Origin><Source>ReferenceFrame</Source><FeatureName></FeatureName></Origin><PrimaryAxis><DefinedDirection>+Z</DefinedDirection><Source>ReferenceFrame</Source><SourceDirection>+Z</SourceDirection><FeatureName></FeatureName></PrimaryAxis><SecondaryAxis><DefinedDirection>+X</DefinedDirection><Source>ReferenceFrame</Source><SourceDirection>+X</SourceDirection><FeatureName></FeatureName></SecondaryAxis></Value></Frame></Frames>  MarkerShape=Sphere  MarkerSize=10  GraphicType=FromGeometry  InertiaType=Custom  Mass=1300  MassUnits=kg  MomentsOfInertia=[1100 1100 1100]  MomentsOfInertiaUnits=kg*m^2  GraphicOpacity=0.6  ProductsOfInertia=[0 0 0]  ProductsOfInertiaUnits=kg*m^2  GraphicShininess=75  GraphicSpecularColor=[0.5 0.5 0.5 1.0]  GraphicVisPropType=SimpleVisualProperties
  Rigid Transform2 : sm_lib/Frames and Transforms/Rigid Transform  TranslationMethod=Cartesian  TranslationStandardOffset=0  TranslationLengthUnit=m  TranslationStandardAxis=+Z  TranslationCartesianOffset=[xref-0.75 0 zref-0.9+1]  TranslationROffset=0  TranslationROffsetUnits=m  TranslationZOffset=0  TranslationZOffsetUnits=m  TranslationThetaOffset=0  TranslationThetaOffsetUnits=deg  RotationMethod=None  RotationAngleUnits=deg  RotationStandardAxis=+Z  RotationAngle=0.0  RotationArbitraryAxis=[0 0 1]  FollAlignAxisA=+X  BaseAlignAxisA=+Y  FollAlignAxisB=+Y  BaseAlignAxisB=+Z  RotationSequenceAxes=FollowerAxes  RotationSequence=XYX  RotationSequenceAngles=[0 0 0]  RotationSequenceAnglesUnits=deg  RotationMatrix=[1 0 0; 0 1 0; 0 0 1]
  Subsystem : Subsystem  Commented=on
      mask Display: disp('Cabin CAD Model')
  Chassis : PMIOPort  Side=Right
  connections:
  Rigid Transform2/RConn1 -- Brick Solid/RConn1
  Chassis/RConn1 -- Rigid Transform2/LConn1
  Subsystem/LConn1 -- Brick Solid/LConn1
